simulink model "Dual_Boost_71V_GEO_PO"  (R2021a)
settings: Solver=VariableStepAuto  StartTime=0.0  StopTime=0.6  RelTol=1e-3
values from neighbouring files (symbols this model uses):
  Ki = x(1,2)    [hybrid_GEO_PO.m]
  Kp = x(1,1)    [hybrid_GEO_PO.m]
undefined symbols (not defined in the file or in its folder): Acid, Ki1, Kp1, Lead, sigbuilder_block
libraries: spsDiodeLib x6, simulink x6, spsCurrentMeasurementLib x5, spsVoltageMeasurementLib x5, spsSeriesRLCBranchLib x4, spsRMSLib x4, spsPVArrayLib x4, spsIGBTLib x3, dsparch4 x2, pid_lib x2, spsControlledVoltageSourceLib x2, spsBatteryLib x1
settings Model: Creator=Administrator  LastModifiedBy=gany0
settings SolverCC: ZeroCrossAlgorithm=Adaptive  AlgebraicLoopSolver=TrustRegion
settings DataIOCC: ReturnWorkspaceOutputs=off
settings DebuggingCC: IgnoredZcDiagnostic=none  SFMachineParentedDataDiag=warning
settings SFSimCC: CustomCodeUndefinedFunction=UseInterfaceOnly

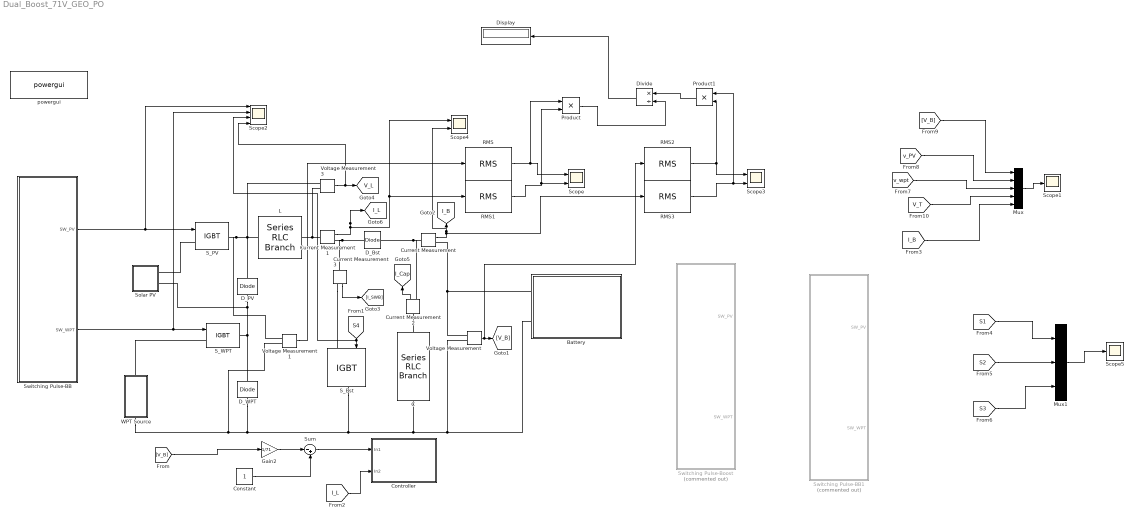
== system Dual_Boost_71V_GEO_PO ==
  "Battery " : Subsystem
  C : spsSeriesRLCBranchLib/Series RLC Branch  LConnTagsString=__new0  RConnTagsString=__new0  BranchType=RC  Resistance=0.01  Inductance=1e-3  SetiL0=off  InitialCurrent=0  Capacitance=1000e-6  Setx0=off  InitialVoltage=120  Measurements=None
  Constant : Constant
  Controller : Subsystem
  Current Measurement{,1..3} (4 alike) : spsCurrentMeasurementLib/Current Measurement  PhasorSimulation=off  OutputType=Complex  PSBequivalent=0
  D_Bst : spsDiodeLib/Diode  Ron=0.001  Lon=0  Vf=0.8  IC=0  UseSnubber=0  Rs=500  Cs=250e-9  Measurements=off
  D_PV : spsDiodeLib/Diode  Ron=0.001  Lon=0  Vf=0.8  IC=0  UseSnubber=0  Rs=500  Cs=250e-9  Measurements=off
  D_WPT : spsDiodeLib/Diode  Ron=0.001  Lon=0  Vf=0.8  IC=0  UseSnubber=0  Rs=500  Cs=250e-9  Measurements=off
  Display : Display
  Divide : Product  Inputs=*/
  Gain2 : Gain  Gain=1/71
  L : spsSeriesRLCBranchLib/Series RLC Branch  LConnTagsString=__new0  RConnTagsString=__new0  BranchType=RL  Resistance=0.01  Inductance=6e-3  SetiL0=off  InitialCurrent=0  Capacitance=1e-6  Setx0=off  InitialVoltage=0  Measurements=None
  Mux : Mux  Inputs=5
  Mux1 : Mux  Inputs=3
  Product : Product
  Product1 : Product
  RMS{,1..3} (4 alike) : spsRMSLib/RMS  TrueRMS=on  Freq=20e3  RMSInit=0  Ts=0
  S_Bst : spsIGBTLib/IGBT  Ron=0.001  Lon=0  Vf=1  Tf=1e-6  Tt=2e-6  IC=0  Rs=1e5  Cs=inf  Measurements=off
  S_PV : spsIGBTLib/IGBT  Ron=0.001  Lon=0  Vf=1  Tf=1e-6  Tt=2e-6  IC=0  Rs=1e5  Cs=inf  Measurements=off
  S_WPT : spsIGBTLib/IGBT  Ron=0.001  Lon=0  Vf=1  Tf=1e-6  Tt=2e-6  IC=0  Rs=1e5  Cs=inf  Measurements=off
  Scope : Scope  NumInputPorts=2
  Scope1 : Scope
  Scope2 : Scope  NumInputPorts=4
  Scope3 : Scope  NumInputPorts=2
  Scope4 : Scope  NumInputPorts=2
  Scope5 : Scope
  Solar PV : Subsystem
  Sum : Sum  Inputs=|-+
  Switching Pulse-BB : Subsystem
  Switching Pulse-BB1 : Subsystem  Commented=on
  Switching Pulse-Boost : Subsystem  Commented=on
  Voltage Measurement : spsVoltageMeasurementLib/Voltage Measurement  PhasorSimulation=off  OutputType=Complex  PSBequivalent=0
  Voltage Measurement1 : spsVoltageMeasurementLib/Voltage Measurement  PhasorSimulation=off  OutputType=Complex  PSBequivalent=0
  Voltage Measurement3 : spsVoltageMeasurementLib/Voltage Measurement  PhasorSimulation=off  OutputType=Complex  PSBequivalent=0
  WPT Source : Subsystem
  powergui : spspowerguiLib/powergui  Priority=1  SimulationMode=Continuous  SampleTime=1/20e3  frequency=60  Iterations=50  frequencyindice=0  Pbase=100e6  ErrMax=1e-4  UnitsV=kV  UnitsW=MW  buscounter=0  FunctionMessages=off  echomessages=off  EnableUseOfTLC=off  CurrentSourceSwitches=off  DisableSnubberDevices=off  DisableRonSwitches=off  DisableVfSwitches=off  DisplayEquations=off  AutomaticDiscreteSolvers=off  SolverType=Tustin/Backward Euler (TBE)  Interpol=off  ExternalGateDelay=off  methode=off  Ts=100  x0status=blocks  SPID=on  SwTol=0  HookPort=off  NonlinearTolerance=0  nMaxIteration=15  ContinueOnMaxIteration=off  RestoreLinks=warning  ResistiveCurrentMeasurement=off  Frange=[0:2:500]  Ylog=off  Xlog=on  ShowGrid=off  save=off  variable=ZData  structure=0  ZoomFFT=off  StartTime=0.0  cycles=1  DisplayStyle=1  fundamental=60  FreqAxis=off  MaxFrequency=1000  frequencyindicesteady=1  RmsSteady=1  display=off
  tag scope: I_B=global, I_Cap=global, I_L=global, V_L=global
  wires:
  Current Measurement1/1 -> [I_L], Scope4/1, RMS1/1
  [S4] -> Scope2/3, S_Bst/1
  Current Measurement3/1 -> [I_SWB]
  Voltage Measurement/1 -> RMS2/1, [V_B]
  Constant/1 -> Sum/2
  Sum/1 -> Controller/1(In1)
  Gain2/1 -> Sum/1
  Mux/1 -> Scope1/1
  Switching Pulse-BB/1(SW_PV) -> Scope2/1, S_PV/1
  Switching Pulse-BB/2(SW_WPT) -> Scope2/2, S_WPT/1
  Current Measurement/1 -> Scope4/2, [I_B], RMS3/1
  Voltage Measurement3/1 -> Scope2/4, [V_L]
  Current Measurement2/1 -> [I_Cap]
  RMS/1 -> Product/1, Scope/1
  RMS1/1 -> Product/2, Scope/2
  RMS3/1 -> Product1/1, Scope3/2
  RMS2/1 -> Product1/2, Scope3/1
  Product/1 -> Divide/2
  Product1/1 -> Divide/1
  Divide/1 -> Display/1
  Voltage Measurement1/1 -> RMS/1
  [V_B] -> Gain2/1
  [V_B] -> Mux/1
  [v_PV] -> Mux/2
  [v_wpt] -> Mux/3
  [V_T] -> Mux/4
  [I_L] -> Controller/2(In2)
  [I_B] -> Mux/5
  Mux1/1 -> Scope5/1
  [S1] -> Mux1/1
  [S2] -> Mux1/2
  [S3] -> Mux1/3
  connections:
  D_Bst/LConn1 -- Current Measurement3/LConn1 -- Current Measurement1/RConn1
  Current Measurement1/LConn1 -- Voltage Measurement3/LConn2 -- L/LConn1
  WPT Source/LConn1 -- Voltage Measurement1/LConn2 -- S_Bst/RConn1 -- "Battery "/LConn2 -- Voltage Measurement/LConn2 -- C/RConn1 -- D_WPT/LConn1
  S_PV/RConn1 -- Voltage Measurement1/LConn1 -- Voltage Measurement3/LConn1 -- D_PV/RConn1 -- L/RConn1
  Current Measurement2/RConn1 -- Current Measurement/LConn1 -- D_Bst/RConn1
  S_WPT/RConn1 -- D_PV/LConn1 -- Solar PV/RConn2 -- D_WPT/RConn1
  Voltage Measurement/LConn1 -- Current Measurement/RConn1 -- "Battery "/LConn1
  Current Measurement3/RConn1 -- S_Bst/LConn1
  Current Measurement2/LConn1 -- C/LConn1
  S_PV/LConn1 -- Solar PV/RConn1
  WPT Source/RConn1 -- S_WPT/LConn1

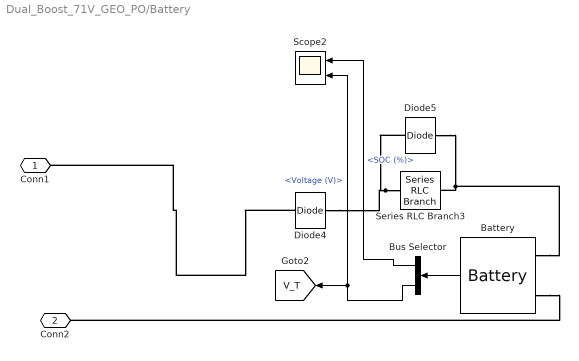
== system Dual_Boost_71V_GEO_PO/Battery  ==
  Battery : spsBatteryLib/Battery  BatType=Lead-Acid  ShowTempParam=off  ThermalPreset=no  ShowAgeParam=off  NomV=60  NomQ=6  SOC=55  Batt_Tr=1  PresetModel=on  MaxQ=6.25  MinV=45  FullV=65.3289  Dis_rate=1.2  R=0.1  Normal_OP=1.8617  expZone="[61.0855         0.02]"  current=[6.5 13 32.5]  Units=Time  Tci=20  NomT=20  T2=-30  MaxQ2=4.8  FullV2=7.1  Normal_OP2=5.655  expZone2="[6.58           1]"  Rca=0.6  ti=2000  Dp=0  Neq0=0  Tsim=1e6  Ta1=25  Qeol=5.4*0.9  Reol=0.013333*1.2  Char_age=[2.3478, 3]  Dis_age=[2.3478, 10]  N1=1500  N2=10500  N3=1000  N4=1400  Ta2=45  N5=950
  Bus Selector : BusSelector  OutputSignals=SOC (%),Voltage (V)
  Diode4 : spsDiodeLib/Diode  Ron=0.001  Lon=0  Vf=0.8  IC=0  UseSnubber=0  Rs=500  Cs=250e-9  Measurements=off
  Diode5 : spsDiodeLib/Diode  Ron=0.001  Lon=0  Vf=0.8  IC=0  UseSnubber=0  Rs=500  Cs=250e-9  Measurements=off
  Scope2 : Scope  NumInputPorts=2
  Series RLC Branch3 : spsSeriesRLCBranchLib/Series RLC Branch  LConnTagsString=__new0  RConnTagsString=__new0  BranchType=RL  Resistance=1  Inductance=1e-3  SetiL0=off  InitialCurrent=0  Capacitance=1e-6  Setx0=off  InitialVoltage=0  Measurements=None
  Conn1 : PMIOPort  Side=Left
  Conn2 : PMIOPort  Port=2  Side=Left
  tag scope: V_T=global
  wires:
  Bus Selector/2 -> Scope2/2, [V_T]  "<Voltage (V)>"
  Battery/1 -> Bus Selector/1
  Bus Selector/1 -> Scope2/1  "<SOC (%)>"
  connections:
  Series RLC Branch3/LConn1 -- Diode4/RConn1 -- Diode5/RConn1
  Diode4/LConn1 -- Conn1/RConn1
  Diode5/LConn1 -- Battery/LConn1 -- Series RLC Branch3/RConn1
  Battery/LConn2 -- Conn2/RConn1

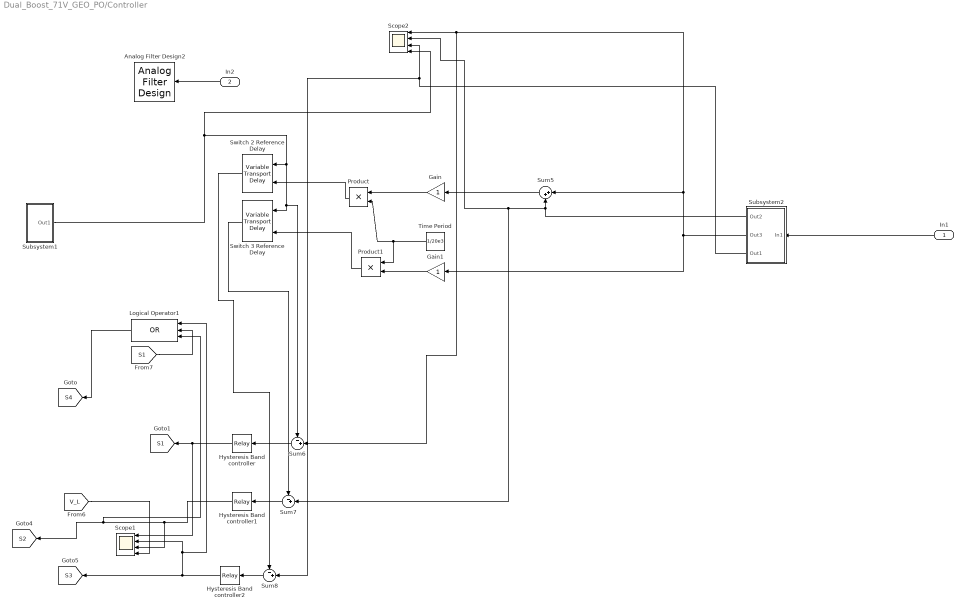
== system Dual_Boost_71V_GEO_PO/Controller ==
  In1 : Inport
  In2 : Inport  Port=2
  Analog Filter Design2 : dsparch4/Analog Filter Design  method=Butterworth  filttype=Lowpass  N=2  Wlo=20e3*3.14*2  Whi=80  Rp=2  Rs=40
  Gain : Gain
  Gain1 : Gain
  Hysteresis Band controller : Relay  OnSwitchValue=0.0001  OffSwitchValue=-0.000001
  Hysteresis Band controller1 : Relay  OnSwitchValue=0.0001  OffSwitchValue=-0.000001
  Hysteresis Band controller2 : Relay  OnSwitchValue=0.0001  OffSwitchValue=-0.000001
  Logical Operator1 : Logic  Operator=OR  Inputs=3  AllPortsSameDT=off  OutDataTypeStr=boolean
  Product : Product
  Product1 : Product
  Scope1 : Scope  NumInputPorts=4
  Scope2 : Scope  NumInputPorts=4
  Subsystem1 : Subsystem
  Subsystem2 : Subsystem
  Sum5 : Sum  Inputs=|++
  Sum6 : Sum  Inputs=-+|
  Sum7 : Sum  Inputs=-+|
  Sum8 : Sum  Inputs=-+|
  Switch 2 Reference Delay : VariableTransportDelay  MaximumDelay=10
  Switch 3 Reference Delay : VariableTransportDelay  MaximumDelay=10
  Time Period : Constant  Value=1/20e3
  tag scope: S1=global, S2=global, S3=global, S4=global
  wires:
  Time Period/1 -> Product/2, Product1/1
  Switch 2 Reference Delay/1 -> Sum8/1
  Logical Operator1/1 -> [S4]
  Hysteresis Band controller2/1 -> [S3], Scope1/2, Logical Operator1/1
  Hysteresis Band controller1/1 -> Scope1/3, Logical Operator1/3, [S2]
  [V_L] -> Scope1/4
  Hysteresis Band controller/1 -> Scope1/1, [S1]
  Switch 3 Reference Delay/1 -> Sum7/1
  [S1] -> Logical Operator1/2
  Sum5/1 -> Gain/1
  Subsystem2/2(Out3) -> Gain1/1, Sum5/1, Scope2/1, Sum6/2
  Product/1 -> Switch 2 Reference Delay/2
  Product1/1 -> Switch 3 Reference Delay/2
  Sum6/1 -> Hysteresis Band controller/1
  Sum7/1 -> Hysteresis Band controller1/1
  Sum8/1 -> Hysteresis Band controller2/1
  Subsystem2/1(Out2) -> Scope2/2, Sum7/2, Sum5/2
  Subsystem2/3(Out1) -> Scope2/3, Sum8/2
  In1/1 -> Subsystem2/1(In1)
  Gain/1 -> Product/1
  Gain1/1 -> Product1/2
  Subsystem1/1(Out1) -> Scope2/4, Sum6/1, Switch 3 Reference Delay/1, Switch 2 Reference Delay/1
  In2/1 -> Analog Filter Design2/1

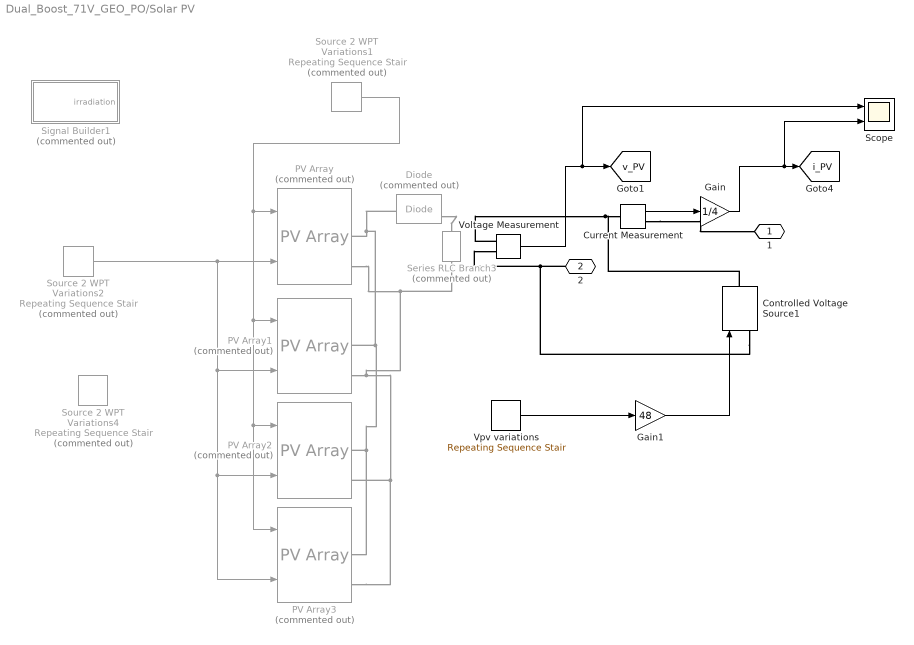
== system Dual_Boost_71V_GEO_PO/Solar PV ==
  Controlled Voltage Source1 : spsControlledVoltageSourceLib/Controlled Voltage Source  Initialize=on  Source_Type=DC  Amplitude=0  Phase=0  Frequency=0  Measurements=None
  Current Measurement : spsCurrentMeasurementLib/Current Measurement  PhasorSimulation=off  OutputType=Complex  PSBequivalent=0
  Diode : spsDiodeLib/Diode  Commented=on  Ron=0.001  Lon=0  Vf=0.8  IC=0  UseSnubber=0  Rs=500  Cs=250e-9  Measurements=on
  Gain : Gain  Gain=1/4
  Gain1 : Gain  Gain=48
  PV Array{,1..3} (4 alike) : spsPVArrayLib/PV Array  Commented=on  Npar=10  Nser=1  PlotType=array @ 1000 W/m2 & specified temperatures  S_vec="[ 1000  500  100 ]"  Temp_C_vec="[ 45 25  ]"  ModuleName=Advance Solar Hydro Wind Power API-150  PlotWhenSelected=off  Pm=150.075  Ncell=72  Voc=41.8  Isc=5.05  Vm=34.5  Im=4.35  beta_Voc_pc=-0.419  alpha_Isc_pc=0.096  beta_Voc=-0.17514  alpha_Isc=0.004848  IL=5.0762  I0=1.155e-09  nI=1.0233  Rsh=71.9537  Rs=0.37337  RobustModel=off  RobustCellTemperature=313.3991  BAL=off  Tc=1e-6  Tfilter=5e-5
  Scope : Scope  NumInputPorts=2
  Series RLC Branch3 : spsSeriesRLCBranchLib/Series RLC Branch  Commented=on  LConnTagsString=__new0  RConnTagsString=__new0  BranchType=C  Resistance=0.01  Inductance=1e-3  SetiL0=off  InitialCurrent=0  Capacitance=1000e-6  Setx0=off  InitialVoltage=120  Measurements=None
  Signal Builder1 : Subsystem  Tag=STV Subsys  Commented=on  LoadFcn=sigbuilder_block('load');  StartFcn=sigbuilder_block('start');  StopFcn=sigbuilder_block('stop');  ClipboardFcn=sigbuilder_block('clipboard');  mask(Sigbuilder block){tuvar=[0:10]}
      mask help: Simulink:masks:SigbuilderBlock_MD
      mask init:
      | if ~strcmp(get_param(bdroot(gcbh),'SimulationStatus'),'stopped') tuvar = sigbuilder_block('maskInit'); end
      settings: CopyFcn=sigbuilder_block('copy');  DeleteFcn=sigbuilder_block('delete');  ModelCloseFcn=sigbuilder_block('modelClose');  PreSaveFcn=sigbuilder_block('preSave');  PauseFcn=sigbuilder_block('pause');  ContinueFcn=sigbuilder_block('continue');  NameChangeFcn=sigbuilder_block('namechange');  OpenFcn=sigbuilder_block('open',[193.2 120.6 550.8 400.2 ]);  CloseFcn=sigbuilder_block('close');
      mask Display: plot(0, 0, 100, 100,[2, 2, 32, 32, 2], [68, 8, 8, 68, 68],[32, 2], [38, 38], [32, 19, 2],[53, 60, 44], [32, 17, 17, 2],[16, 16, 31, 31]);txt = getActiveGroup(gcbh);text(2, 100, txt,'verticalAlignment', 'top');
  Source 2 WPT Variations1 : simulink/Sources/Repeating Sequence Stair  Commented=on  OutValues=[450 500 600 650 700 850 950 950 900 800 750 600 400]  tsamp=1  OutMin=[]  OutMax=[]  OutDataTypeStr=double  OutputDataTypeScalingMode=double  OutDataType=fixdt(0,8)  ConRadixGroup=Best Precision: Vector-wise  OutScaling=2^-12
  Source 2 WPT Variations2 : simulink/Sources/Repeating Sequence Stair  Commented=on  OutValues=[25 26 27 30 32 33 37 35 31 28 24]  tsamp=1  OutMin=[]  OutMax=[]  OutDataTypeStr=double  OutputDataTypeScalingMode=double  OutDataType=fixdt(0,8)  ConRadixGroup=Best Precision: Vector-wise  OutScaling=2^-12
  Source 2 WPT Variations4 : simulink/Sources/Repeating Sequence Stair  Commented=on  OutValues=[1 0.8 0.9 1.1 1.05 1.0 1 0.95 1.2 1]  tsamp=1  OutMin=[]  OutMax=[]  OutDataTypeStr=double  OutputDataTypeScalingMode=double  OutDataType=fixdt(0,8)  ConRadixGroup=Best Precision: Vector-wise  OutScaling=2^-12
  Voltage Measurement : spsVoltageMeasurementLib/Voltage Measurement  PhasorSimulation=off  OutputType=Complex  PSBequivalent=0
  Vpv variations : simulink/Sources/Repeating Sequence Stair  OutValues=[1 1.2 0.75]  tsamp=0.2  OutMin=[]  OutMax=[]  OutDataTypeStr=double  OutputDataTypeScalingMode=double  OutDataType=fixdt(0,8)  ConRadixGroup=Best Precision: Vector-wise  OutScaling=2^-12
  1 : PMIOPort  Side=Right
  2 : PMIOPort  Port=2  Side=Right
  tag scope: i_PV=global, v_PV=global
  wires:
  Source 2 WPT Variations2/1 -> PV Array3/2, PV Array2/2, PV Array1/2, PV Array/2
  Source 2 WPT Variations1/1 -> PV Array3/1, PV Array2/1, PV Array1/1, PV Array/1
  Vpv variations/1 -> Gain1/1
  Gain1/1 -> Controlled Voltage Source1/1
  Voltage Measurement/1 -> Scope/1, [v_PV]
  Current Measurement/1 -> Gain/1
  Gain/1 -> Scope/2, [i_PV]
  connections:
  Voltage Measurement/LConn1 -- Controlled Voltage Source1/RConn1 -- Current Measurement/LConn1
  Current Measurement/RConn1 -- 1/RConn1
  PV Array3/RConn1 -- PV Array/RConn1 -- Diode/LConn1 -- PV Array1/RConn1 -- PV Array2/RConn1
  PV Array1/RConn2 -- PV Array3/RConn2 -- PV Array2/RConn2 -- Series RLC Branch3/RConn1 -- PV Array/RConn2
  Diode/RConn1 -- Series RLC Branch3/LConn1
  2/RConn1 -- Controlled Voltage Source1/LConn1 -- Voltage Measurement/LConn2

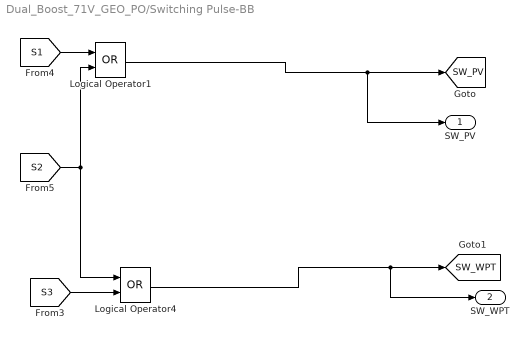
== system Dual_Boost_71V_GEO_PO/Switching Pulse-BB ==
  Logical Operator1 : Logic  Operator=OR  AllPortsSameDT=off  OutDataTypeStr=boolean
  Logical Operator4 : Logic  Operator=OR  AllPortsSameDT=off  OutDataTypeStr=boolean
  SW_PV : Outport
  SW_WPT : Outport  Port=2
  tag scope: SW_PV=global, SW_WPT=global
  wires:
  Logical Operator4/1 -> [SW_WPT], SW_WPT/1
  Logical Operator1/1 -> [SW_PV], SW_PV/1
  [S3] -> Logical Operator4/2
  [S1] -> Logical Operator1/1
  [S2] -> Logical Operator1/2, Logical Operator4/1

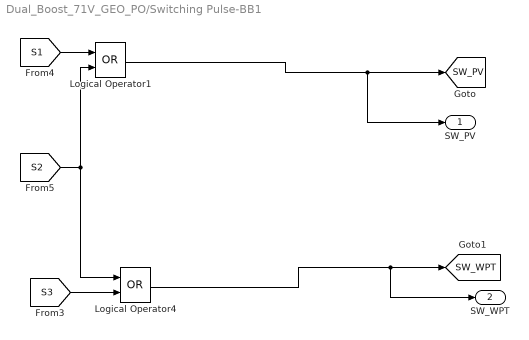
== system Dual_Boost_71V_GEO_PO/Switching Pulse-BB1 ==
  Logical Operator1 : Logic  Operator=OR  AllPortsSameDT=off  OutDataTypeStr=boolean
  Logical Operator4 : Logic  Operator=OR  AllPortsSameDT=off  OutDataTypeStr=boolean
  SW_PV : Outport
  SW_WPT : Outport  Port=2
  tag scope: SW_PV=global, SW_WPT=global
  wires:
  Logical Operator4/1 -> [SW_WPT], SW_WPT/1
  Logical Operator1/1 -> [SW_PV], SW_PV/1
  [S3] -> Logical Operator4/2
  [S1] -> Logical Operator1/1
  [S2] -> Logical Operator1/2, Logical Operator4/1

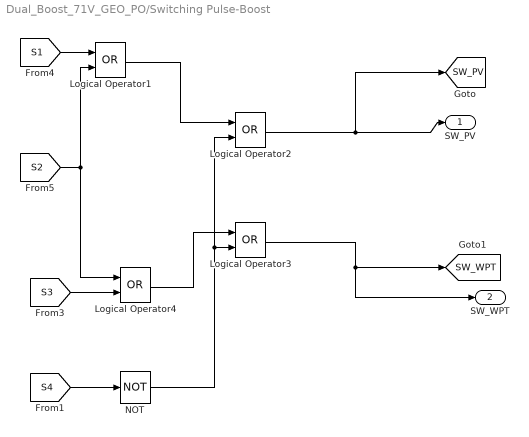
== system Dual_Boost_71V_GEO_PO/Switching Pulse-Boost ==
  Logical Operator{1..4} (4 alike) : Logic  Operator=OR  AllPortsSameDT=off  OutDataTypeStr=boolean
  NOT : Logic  Operator=NOT  IconShape=distinctive  AllPortsSameDT=off  OutDataTypeStr=boolean
  SW_PV : Outport
  SW_WPT : Outport  Port=2
  tag scope: SW_PV=global, SW_WPT=global
  wires:
  [S3] -> Logical Operator4/2
  [S1] -> Logical Operator1/1
  [S2] -> Logical Operator1/2, Logical Operator4/1
  [S4] -> NOT/1
  Logical Operator1/1 -> Logical Operator2/1
  Logical Operator4/1 -> Logical Operator3/1
  NOT/1 -> Logical Operator3/2, Logical Operator2/2
  Logical Operator2/1 -> SW_PV/1, [SW_PV]
  Logical Operator3/1 -> SW_WPT/1, [SW_WPT]

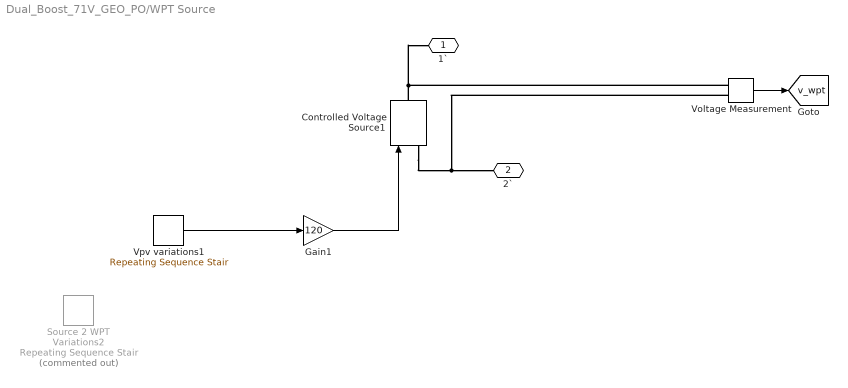
== system Dual_Boost_71V_GEO_PO/WPT Source ==
  Controlled Voltage Source1 : spsControlledVoltageSourceLib/Controlled Voltage Source  Initialize=on  Source_Type=DC  Amplitude=0  Phase=0  Frequency=0  Measurements=None
  Gain1 : Gain  Gain=120
  Source 2 WPT Variations2 : simulink/Sources/Repeating Sequence Stair  Commented=on  OutValues=[1 0.9 1.05 1.0 1 0.95 1.2 1]  tsamp=1  OutMin=[]  OutMax=[]  OutDataTypeStr=double  OutputDataTypeScalingMode=double  OutDataType=fixdt(0,8)  ConRadixGroup=Best Precision: Vector-wise  OutScaling=2^-12
  Voltage Measurement : spsVoltageMeasurementLib/Voltage Measurement  PhasorSimulation=off  OutputType=Complex  PSBequivalent=0
  Vpv variations1 : simulink/Sources/Repeating Sequence Stair  OutValues=[1 1.08 0.9]  tsamp=0.2  OutMin=[]  OutMax=[]  OutDataTypeStr=double  OutputDataTypeScalingMode=double  OutDataType=fixdt(0,8)  ConRadixGroup=Best Precision: Vector-wise  OutScaling=2^-12
  1` : PMIOPort  Side=Right
  2` : PMIOPort  Port=2  Side=Left
  tag scope: v_wpt=global
  wires:
  Gain1/1 -> Controlled Voltage Source1/1
  Vpv variations1/1 -> Gain1/1
  Voltage Measurement/1 -> [v_wpt]
  connections:
  Controlled Voltage Source1/LConn1 -- Voltage Measurement/LConn2 -- 2`/RConn1
  Controlled Voltage Source1/RConn1 -- 1`/RConn1 -- Voltage Measurement/LConn1

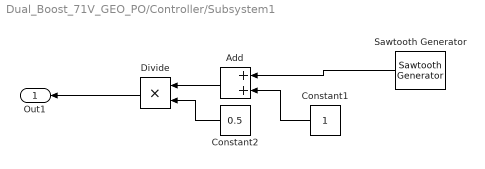
== system Dual_Boost_71V_GEO_PO/Controller/Subsystem1 ==
  Add : Sum
  Constant1 : Constant
  Constant2 : Constant  Value=0.5
  Divide : Product  Inputs=**
  Sawtooth Generator : spsSawtoothGeneratorLib/Sawtooth Generator  Freq=20e3  Phase=0  Ts=0
  Out1 : Outport
  wires:
  Sawtooth Generator/1 -> Add/1
  Constant1/1 -> Add/2
  Add/1 -> Divide/1
  Constant2/1 -> Divide/2
  Divide/1 -> Out1/1

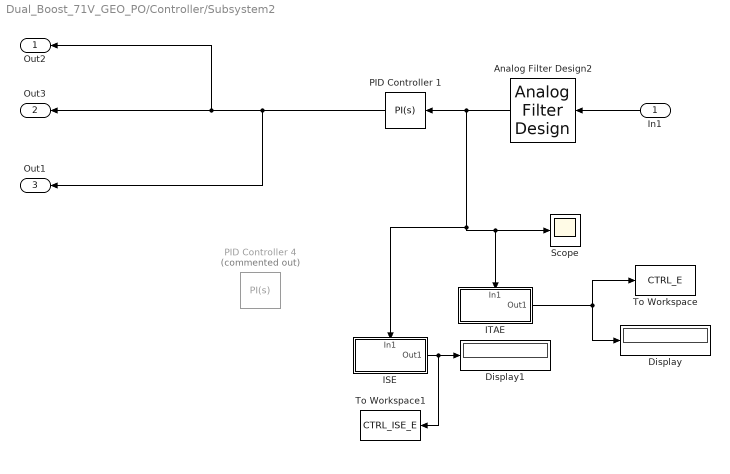
== system Dual_Boost_71V_GEO_PO/Controller/Subsystem2 ==
  In1 : Inport
  Analog Filter Design2 : dsparch4/Analog Filter Design  method=Butterworth  filttype=Lowpass  N=2  Wlo=20e3*3.14*2  Whi=80  Rp=2  Rs=40
  Display : Display
  Display1 : Display
  ISE : Subsystem
      mask help:
      | ITAE performance index
      |
      | output = int t|input| dt
      settings: PortSchema="{\"entries\":[{\"content\":{\"sides\":[{\"content\":{\"connectorIds\":[]},\"type\":\"ConnectorPlacement.EquallySpacedRectSide\",\"uuid\":\"dc380c11-ed8a-4907-ad1a-93a594419ac9\"},{\"content\":{\"connectorIds\":[\"Out1\"],\"side\":\"RIGHT\"},\"type\":\"ConnectorPlacement.EquallySpacedRectSide\",\"uuid\":\"4ddb2573-2ea1-4c8e-bb30-822497078c6f\"},{\"content\":{\"connectorIds\":[\"In1\"],\"side\":\"TOP\"},\"type\":\"ConnectorPlacement.EquallySpacedRectSide\",\"uuid\":\"63f9bd1d-f55b-4ceb-8617-4a3fd5d1e5a5\"}]},\"type\":\"ConnectorPlacement.EquallySpacedConnector\",\"uuid\":\"09ea5f2b-c71c-4206-bf03-fbcb7ad0d6a0\"}],\"packageUris\":[\"http://schema.mathworks.com/mf0/Connector/R2020b\"],\"version\":\"1.0\"}"
      mask Display:
      | disp('ISE')
      | port_label('input',1,'e')
      | port_label('output',1,'ise')
  ITAE : Subsystem
      mask help:
      | ITAE performance index
      |
      | output = int t|input| dt
      settings: PortSchema="{\"entries\":[{\"content\":{\"sides\":[{\"content\":{\"connectorIds\":[]},\"type\":\"ConnectorPlacement.EquallySpacedRectSide\",\"uuid\":\"dc380c11-ed8a-4907-ad1a-93a594419ac9\"},{\"content\":{\"connectorIds\":[\"Out1\"],\"side\":\"RIGHT\"},\"type\":\"ConnectorPlacement.EquallySpacedRectSide\",\"uuid\":\"4ddb2573-2ea1-4c8e-bb30-822497078c6f\"},{\"content\":{\"connectorIds\":[\"In1\"],\"side\":\"TOP\"},\"type\":\"ConnectorPlacement.EquallySpacedRectSide\",\"uuid\":\"63f9bd1d-f55b-4ceb-8617-4a3fd5d1e5a5\"}]},\"type\":\"ConnectorPlacement.EquallySpacedConnector\",\"uuid\":\"09ea5f2b-c71c-4206-bf03-fbcb7ad0d6a0\"}],\"packageUris\":[\"http://schema.mathworks.com/mf0/Connector/R2020b\"],\"version\":\"1.0\"}"
      mask Display:
      | disp('ITAE')
      | port_label('input',1,'e')
      | port_label('output',1,'itae')
  PID Controller 1 : pid_lib/PID Controller  Controller=PI  Form=Parallel  TimeDomain=Continuous-time  UseExternalTs=off  SampleTime=-1  IntegratorMethod=Forward Euler  FilterMethod=Forward Euler  ControllerParametersSource=internal  P=Kp  I=Ki  D=0  UseFilter=on  N=400  TunerSelectOption=Transfer Function Based (PID Tuner App)  InitialConditionSource=internal  InitialConditionForIntegrator=0  InitialConditionForFilter=0  DifferentiatorICPrevScaledInput=0  ExternalReset=none  TrackingMode=off  Kt=1  LimitOutput=off  SatLimitsSource=internal  UpperSaturationLimit=inf  LowerSaturationLimit=-inf  LinearizeAsGain=on  AntiWindupMode=back-calculation  Kb=1  POutMin=[]  POutMax=[]  IOutMin=[]  IOutMax=[]  DOutMin=[]  DOutMax=[]  NOutMin=[]  NOutMax=[]  SumOutMin=[]  SumOutMax=[]  SaturationOutMin=[]  SaturationOutMax=[]  PParamMin=[]  PParamMax=[]  IParamMin=[]  IParamMax=[]  DParamMin=[]  DParamMax=[]  NParamMin=[]  NParamMax=[]  KbParamMin=[]  KbParamMax=[]  KtParamMin=[]  KtParamMax=[]  KbOutMin=[]  KbOutMax=[]  KtOutMin=[]  KtOutMax=[]  IntegratorOutMin=[]  IntegratorOutMax=[]  FilterOutMin=[]  FilterOutMax=[]  SumI1OutMin=[]  SumI1OutMax=[]  SumI2OutMin=[]  SumI2OutMax=[]  SumI3OutMin=[]  SumI3OutMax=[]  SumI4OutMin=[]  SumI4OutMax=[]  SumDOutMin=[]  SumDOutMax=[]  DifferentiatorOutMin=[]  DifferentiatorOutMax=[]  FilterDiffOutCoefMin=[]  FilterDiffOutCoefMax=[]  ReciprocalOutMin=[]  ReciprocalOutMax=[]  SumDenOutMin=[]  SumDenOutMax=[]  SumNumOutMin=[]  SumNumOutMax=[]  DivideOutMin=[]  DivideOutMax=[]  UdiffTsProdOutMin=[]  UdiffTsProdOutMax=[]  NTsProdOutMin=[]  NTsProdOutMax=[]  UintegralTsProdOutMin=[]  UintegralTsProdOutMax=[]  UngainTsProdOutMin=[]  UngainTsProdOutMax=[]  IntegratorContinuousStateAttributes=''  IntegratorStateMustResolveToSignalObject=off  IntegratorRTWStateStorageClass=Auto  FilterContinuousStateAttributes=''  FilterStateMustResolveToSignalObject=off  FilterRTWStateStorageClass=Auto  ParallelPVariant=InternalParameters  IdealPVariant=Disabled  IVariant=InternalParameters  DVariant=Disabled  IntegratorVariant=Continuous  SatVariant=Disabled  AWVariant=Passthrough  PCopyVariant=Disabled  TRVariant=Disabled  FdbkBlocksVariant=Forward  IdealPFdbkVariant=Disabled  SatFdbkVariant=Disabled  DerivativeFilterVariant=Disabled  NVariant=Disabled  NCopyVariant=Disabled_SignalSpec  FilterICVariant=Disabled  IntegratorICVariant=InternalICs  ExternalResetVariant=Disabled  TRSumVariant=Passthrough  SumFdbkVariant=Disabled  SumVariant=Sum_PI  TsampFilterVariant=InternalTs  TsampNgainVariant=Passthrough  TsampIntegralVariant=Passthrough  ExternalSaturationOutDataTypeStr=Inherit: Same as second input
  PID Controller 4 : pid_lib/PID Controller  Commented=on  Controller=PI  Form=Parallel  TimeDomain=Continuous-time  UseExternalTs=off  SampleTime=-1  IntegratorMethod=Forward Euler  FilterMethod=Forward Euler  ControllerParametersSource=internal  P=Kp1  I=Ki1  D=0.001  UseFilter=on  N=100  TunerSelectOption=Transfer Function Based (PID Tuner App)  InitialConditionSource=internal  InitialConditionForIntegrator=0  InitialConditionForFilter=0  DifferentiatorICPrevScaledInput=0  ExternalReset=none  TrackingMode=off  Kt=1  LimitOutput=off  SatLimitsSource=internal  UpperSaturationLimit=inf  LowerSaturationLimit=-inf  LinearizeAsGain=on  AntiWindupMode=back-calculation  Kb=1  POutMin=[]  POutMax=[]  IOutMin=[]  IOutMax=[]  DOutMin=[]  DOutMax=[]  NOutMin=[]  NOutMax=[]  SumOutMin=[]  SumOutMax=[]  SaturationOutMin=[]  SaturationOutMax=[]  PParamMin=[]  PParamMax=[]  IParamMin=[]  IParamMax=[]  DParamMin=[]  DParamMax=[]  NParamMin=[]  NParamMax=[]  KbParamMin=[]  KbParamMax=[]  KtParamMin=[]  KtParamMax=[]  KbOutMin=[]  KbOutMax=[]  KtOutMin=[]  KtOutMax=[]  IntegratorOutMin=[]  IntegratorOutMax=[]  FilterOutMin=[]  FilterOutMax=[]  SumI1OutMin=[]  SumI1OutMax=[]  SumI2OutMin=[]  SumI2OutMax=[]  SumI3OutMin=[]  SumI3OutMax=[]  SumI4OutMin=[]  SumI4OutMax=[]  SumDOutMin=[]  SumDOutMax=[]  DifferentiatorOutMin=[]  DifferentiatorOutMax=[]  FilterDiffOutCoefMin=[]  FilterDiffOutCoefMax=[]  ReciprocalOutMin=[]  ReciprocalOutMax=[]  SumDenOutMin=[]  SumDenOutMax=[]  SumNumOutMin=[]  SumNumOutMax=[]  DivideOutMin=[]  DivideOutMax=[]  UdiffTsProdOutMin=[]  UdiffTsProdOutMax=[]  NTsProdOutMin=[]  NTsProdOutMax=[]  UintegralTsProdOutMin=[]  UintegralTsProdOutMax=[]  UngainTsProdOutMin=[]  UngainTsProdOutMax=[]  IntegratorContinuousStateAttributes=''  IntegratorStateMustResolveToSignalObject=off  IntegratorRTWStateStorageClass=Auto  FilterContinuousStateAttributes=''  FilterStateMustResolveToSignalObject=off  FilterRTWStateStorageClass=Auto  ParallelPVariant=InternalParameters  IdealPVariant=Disabled  IVariant=InternalParameters  DVariant=Disabled  IntegratorVariant=Continuous  SatVariant=Disabled  AWVariant=Passthrough  PCopyVariant=Disabled  TRVariant=Disabled  FdbkBlocksVariant=Forward  IdealPFdbkVariant=Disabled  SatFdbkVariant=Disabled  DerivativeFilterVariant=Disabled  NVariant=Disabled  NCopyVariant=Disabled_SignalSpec  FilterICVariant=Disabled  IntegratorICVariant=InternalICs  ExternalResetVariant=Disabled  TRSumVariant=Passthrough  SumFdbkVariant=Disabled  SumVariant=Sum_PI  TsampFilterVariant=InternalTs  TsampNgainVariant=Passthrough  TsampIntegralVariant=Passthrough  ExternalSaturationOutDataTypeStr=Inherit: Same as second input
  Scope : Scope
  To Workspace : ToWorkspace  VariableName=CTRL_E  SampleTime=-1
      settings: MaxDataPoints=1  Save2DSignal=2-D array (concatenate along first dimension)
  To Workspace1 : ToWorkspace  VariableName=CTRL_ISE_E  SampleTime=-1
      settings: MaxDataPoints=1  Save2DSignal=2-D array (concatenate along first dimension)
  Out2 : Outport
  Out3 : Outport  Port=2
  Out1 : Outport  Port=3
  wires:
  In1/1 -> Analog Filter Design2/1
  ITAE/1(Out1) -> To Workspace/1, Display/1
  Analog Filter Design2/1 -> PID Controller 1/1, ISE/1(In1), ITAE/1(In1), Scope/1
  ISE/1(Out1) -> To Workspace1/1, Display1/1
  PID Controller 1/1 -> Out1/1, Out2/1, Out3/1

== system Dual_Boost_71V_GEO_PO/Solar PV/Signal Builder1 ==
  Demux : Demux  Tag=STV Demux  Outputs=1
      settings: DisplayOption=none
  FromWs : FromWorkspace  Tag=STV FromWs  VariableName=tuvar
      SigBuilderData=|
      | common.afterFinalStr = 'Extrapolate'
      | common.sampleTime = 0
      | dataSet.timeRange = [0 4]
      | dataSet.name = 'Group 1'
      | sbobj.Groups.Name = 'Group 1'
      | sbobj.Groups.Signals.Name = 'irradiation'
      | sbobj.Groups.Signals.XData = [0 0.004 0.008 0.012 0.016 0.02 0.024 0.028 0.032 0.036 0.04 0.044 ... (1000 elements, 1x1000)]
      | sbobj.Groups.Signals.YData = [2.7183440665 2.7183440665 2.7183440665 2.7183440665 2.7183440665 2.7183440665 2.7183440665 2.7183440665 2.7183440665 2.71833264456 2.71833264456 2.71833264456 ... (1000 elements, 1x1000)]
      | sbobj.Groups.TimeRange = [0 4]
  irradiation : Outport  Tag=STV Outport
  wires:
  FromWs/1 -> Demux/1
  Demux/1 -> irradiation/1

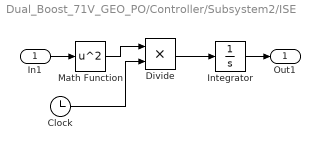
== system Dual_Boost_71V_GEO_PO/Controller/Subsystem2/ISE ==
  In1 : Inport
  Clock : Clock
  Divide : Product  Inputs=**
  Integrator : Integrator
  Math Function : Math  Operator=square  SaturateOnIntegerOverflow=on
  Out1 : Outport
  wires:
  Integrator/1 -> Out1/1
  In1/1 -> Math Function/1
  Divide/1 -> Integrator/1
  Math Function/1 -> Divide/1
  Clock/1 -> Divide/2

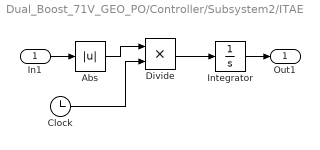
== system Dual_Boost_71V_GEO_PO/Controller/Subsystem2/ITAE ==
  In1 : Inport
  Abs : Abs
  Clock : Clock
  Divide : Product  Inputs=**
  Integrator : Integrator
  Out1 : Outport
  wires:
  Integrator/1 -> Out1/1
  In1/1 -> Abs/1
  Divide/1 -> Integrator/1
  Abs/1 -> Divide/1
  Clock/1 -> Divide/2
